simulink model "TEModel_random"  (Simulink 8.3)
settings: Solver=ode1  SolverMode=SingleTasking  StartTime=0.0  StopTime=72  FixedStep=Ts_base  MaxStep=Ts_base  MinStep=1e-6  RelTol=1e-6
PreLoadFcn:
  | initModel
StopFcn:
  | TEplot
undefined symbols (not defined in the file): Ts_base, Ts_save
libraries: VAlib x28, TElib x18
(part 9 of 9)

== system TEModel_random/TE Plant/xmeas atk block/xmeas3 attack controller/Attack Type Controller/interval forward controller ==
  normal : Inport
  faked : Inport  Port=2
  Impuls : VAlib/Impuls  amplitude=1  duration=duration  delay=start
  Switch : Switch  Criteria=u2 > Threshold
  output : Outport
  wires:
  faked/1 -> Switch/1
  normal/1 -> Switch/3
  Impuls/1 -> Switch/2
  Switch/1 -> output/1

== system TEModel_random/TE Plant/xmeas atk block/xmeas3 attack controller/Attack Type Controller/normal forward controller ==
  normal : Inport
  faked : Inport  Port=2
  Terminator : Terminator
  output : Outport
  wires:
  normal/1 -> output/1
  faked/1 -> Terminator/1

== system TEModel_random/TE Plant/xmeas atk block/xmeas3 attack controller/Attack Type Controller/periodical forward controller ==
  normal : Inport
  faked : Inport  Port=2
  Pulse Generator : DiscretePulseGenerator  PulseType=Time based  Period=duration + start  PulseWidth=100*duration/(duration + start)  PhaseDelay=start
  Switch : Switch  Criteria=u2 > Threshold
  output : Outport
  wires:
  faked/1 -> Switch/1
  normal/1 -> Switch/3
  Pulse Generator/1 -> Switch/2
  Switch/1 -> output/1

== system TEModel_random/TE Plant/xmeas atk block/xmeas3 attack controller/Attack Type Controller/step forward controller ==
  normal : Inport
  faked : Inport  Port=2
  Step : Step  Time=start  SampleTime=0
  Switch : Switch  Criteria=u2 > Threshold
  output : Outport
  wires:
  faked/1 -> Switch/1
  normal/1 -> Switch/3
  Step/1 -> Switch/2
  Switch/1 -> output/1

== system TEModel_random/TE Plant/xmeas atk block/xmeas31 attack controller/Attack Type Controller/interval forward controller ==
  normal : Inport
  faked : Inport  Port=2
  Impuls : VAlib/Impuls  amplitude=1  duration=duration  delay=start
  Switch : Switch  Criteria=u2 > Threshold
  output : Outport
  wires:
  faked/1 -> Switch/1
  normal/1 -> Switch/3
  Impuls/1 -> Switch/2
  Switch/1 -> output/1

== system TEModel_random/TE Plant/xmeas atk block/xmeas31 attack controller/Attack Type Controller/normal forward controller ==
  normal : Inport
  faked : Inport  Port=2
  Terminator : Terminator
  output : Outport
  wires:
  normal/1 -> output/1
  faked/1 -> Terminator/1

== system TEModel_random/TE Plant/xmeas atk block/xmeas31 attack controller/Attack Type Controller/periodical forward controller ==
  normal : Inport
  faked : Inport  Port=2
  Pulse Generator : DiscretePulseGenerator  PulseType=Time based  Period=duration + start  PulseWidth=100*duration/(duration + start)  PhaseDelay=start
  Switch : Switch  Criteria=u2 > Threshold
  output : Outport
  wires:
  faked/1 -> Switch/1
  normal/1 -> Switch/3
  Pulse Generator/1 -> Switch/2
  Switch/1 -> output/1

== system TEModel_random/TE Plant/xmeas atk block/xmeas31 attack controller/Attack Type Controller/step forward controller ==
  normal : Inport
  faked : Inport  Port=2
  Step : Step  Time=start  SampleTime=0
  Switch : Switch  Criteria=u2 > Threshold
  output : Outport
  wires:
  faked/1 -> Switch/1
  normal/1 -> Switch/3
  Step/1 -> Switch/2
  Switch/1 -> output/1

== system TEModel_random/TE Plant/xmeas atk block/xmeas4 attack controller/Attack Type Controller/interval forward controller ==
  normal : Inport
  faked : Inport  Port=2
  Impuls : VAlib/Impuls  amplitude=1  duration=duration  delay=start
  Switch : Switch  Criteria=u2 > Threshold
  output : Outport
  wires:
  faked/1 -> Switch/1
  normal/1 -> Switch/3
  Impuls/1 -> Switch/2
  Switch/1 -> output/1

== system TEModel_random/TE Plant/xmeas atk block/xmeas4 attack controller/Attack Type Controller/normal forward controller ==
  normal : Inport
  faked : Inport  Port=2
  Terminator : Terminator
  output : Outport
  wires:
  normal/1 -> output/1
  faked/1 -> Terminator/1

== system TEModel_random/TE Plant/xmeas atk block/xmeas4 attack controller/Attack Type Controller/periodical forward controller ==
  normal : Inport
  faked : Inport  Port=2
  Pulse Generator : DiscretePulseGenerator  PulseType=Time based  Period=duration + start  PulseWidth=100*duration/(duration + start)  PhaseDelay=start
  Switch : Switch  Criteria=u2 > Threshold
  output : Outport
  wires:
  faked/1 -> Switch/1
  normal/1 -> Switch/3
  Pulse Generator/1 -> Switch/2
  Switch/1 -> output/1

== system TEModel_random/TE Plant/xmeas atk block/xmeas4 attack controller/Attack Type Controller/step forward controller ==
  normal : Inport
  faked : Inport  Port=2
  Step : Step  Time=start  SampleTime=0
  Switch : Switch  Criteria=u2 > Threshold
  output : Outport
  wires:
  faked/1 -> Switch/1
  normal/1 -> Switch/3
  Step/1 -> Switch/2
  Switch/1 -> output/1

== system TEModel_random/TE Plant/xmeas atk block/xmeas40 attack controller/Attack Type Controller/interval forward controller ==
  normal : Inport
  faked : Inport  Port=2
  Impuls : VAlib/Impuls  amplitude=1  duration=duration  delay=start
  Switch : Switch  Criteria=u2 > Threshold
  output : Outport
  wires:
  faked/1 -> Switch/1
  normal/1 -> Switch/3
  Impuls/1 -> Switch/2
  Switch/1 -> output/1

== system TEModel_random/TE Plant/xmeas atk block/xmeas40 attack controller/Attack Type Controller/normal forward controller ==
  normal : Inport
  faked : Inport  Port=2
  Terminator : Terminator
  output : Outport
  wires:
  normal/1 -> output/1
  faked/1 -> Terminator/1

== system TEModel_random/TE Plant/xmeas atk block/xmeas40 attack controller/Attack Type Controller/periodical forward controller ==
  normal : Inport
  faked : Inport  Port=2
  Pulse Generator : DiscretePulseGenerator  PulseType=Time based  Period=duration + start  PulseWidth=100*duration/(duration + start)  PhaseDelay=start
  Switch : Switch  Criteria=u2 > Threshold
  output : Outport
  wires:
  faked/1 -> Switch/1
  normal/1 -> Switch/3
  Pulse Generator/1 -> Switch/2
  Switch/1 -> output/1

== system TEModel_random/TE Plant/xmeas atk block/xmeas40 attack controller/Attack Type Controller/step forward controller ==
  normal : Inport
  faked : Inport  Port=2
  Step : Step  Time=start  SampleTime=0
  Switch : Switch  Criteria=u2 > Threshold
  output : Outport
  wires:
  faked/1 -> Switch/1
  normal/1 -> Switch/3
  Step/1 -> Switch/2
  Switch/1 -> output/1

== system TEModel_random/TE Plant/xmeas atk block/xmeas5 attack controller/Attack Type Controller/interval forward controller ==
  normal : Inport
  faked : Inport  Port=2
  Impuls : VAlib/Impuls  amplitude=1  duration=duration  delay=start
  Switch : Switch  Criteria=u2 > Threshold
  output : Outport
  wires:
  faked/1 -> Switch/1
  normal/1 -> Switch/3
  Impuls/1 -> Switch/2
  Switch/1 -> output/1

== system TEModel_random/TE Plant/xmeas atk block/xmeas5 attack controller/Attack Type Controller/normal forward controller ==
  normal : Inport
  faked : Inport  Port=2
  Terminator : Terminator
  output : Outport
  wires:
  normal/1 -> output/1
  faked/1 -> Terminator/1

== system TEModel_random/TE Plant/xmeas atk block/xmeas5 attack controller/Attack Type Controller/periodical forward controller ==
  normal : Inport
  faked : Inport  Port=2
  Pulse Generator : DiscretePulseGenerator  PulseType=Time based  Period=duration + start  PulseWidth=100*duration/(duration + start)  PhaseDelay=start
  Switch : Switch  Criteria=u2 > Threshold
  output : Outport
  wires:
  faked/1 -> Switch/1
  normal/1 -> Switch/3
  Pulse Generator/1 -> Switch/2
  Switch/1 -> output/1

== system TEModel_random/TE Plant/xmeas atk block/xmeas5 attack controller/Attack Type Controller/step forward controller ==
  normal : Inport
  faked : Inport  Port=2
  Step : Step  Time=start  SampleTime=0
  Switch : Switch  Criteria=u2 > Threshold
  output : Outport
  wires:
  faked/1 -> Switch/1
  normal/1 -> Switch/3
  Step/1 -> Switch/2
  Switch/1 -> output/1

== system TEModel_random/TE Plant/xmeas atk block/xmeas7 attack controller/Attack Type Controller/interval forward controller ==
  normal : Inport
  faked : Inport  Port=2
  Impuls : VAlib/Impuls  amplitude=1  duration=duration  delay=start
  Switch : Switch  Criteria=u2 > Threshold
  output : Outport
  wires:
  faked/1 -> Switch/1
  normal/1 -> Switch/3
  Impuls/1 -> Switch/2
  Switch/1 -> output/1

== system TEModel_random/TE Plant/xmeas atk block/xmeas7 attack controller/Attack Type Controller/normal forward controller ==
  normal : Inport
  faked : Inport  Port=2
  Terminator : Terminator
  output : Outport
  wires:
  normal/1 -> output/1
  faked/1 -> Terminator/1

== system TEModel_random/TE Plant/xmeas atk block/xmeas7 attack controller/Attack Type Controller/periodical forward controller ==
  normal : Inport
  faked : Inport  Port=2
  Pulse Generator : DiscretePulseGenerator  PulseType=Time based  Period=duration + start  PulseWidth=100*duration/(duration + start)  PhaseDelay=start
  Switch : Switch  Criteria=u2 > Threshold
  output : Outport
  wires:
  faked/1 -> Switch/1
  normal/1 -> Switch/3
  Pulse Generator/1 -> Switch/2
  Switch/1 -> output/1

== system TEModel_random/TE Plant/xmeas atk block/xmeas7 attack controller/Attack Type Controller/step forward controller ==
  normal : Inport
  faked : Inport  Port=2
  Step : Step  Time=start  SampleTime=0
  Switch : Switch  Criteria=u2 > Threshold
  output : Outport
  wires:
  faked/1 -> Switch/1
  normal/1 -> Switch/3
  Step/1 -> Switch/2
  Switch/1 -> output/1

== system TEModel_random/TE Plant/xmeas atk block/xmeas8 attack controller/Attack Type Controller/interval forward controller ==
  normal : Inport
  faked : Inport  Port=2
  Impuls : VAlib/Impuls  amplitude=1  duration=duration  delay=start
  Switch : Switch  Criteria=u2 > Threshold
  output : Outport
  wires:
  faked/1 -> Switch/1
  normal/1 -> Switch/3
  Impuls/1 -> Switch/2
  Switch/1 -> output/1

== system TEModel_random/TE Plant/xmeas atk block/xmeas8 attack controller/Attack Type Controller/normal forward controller ==
  normal : Inport
  faked : Inport  Port=2
  Terminator : Terminator
  output : Outport
  wires:
  normal/1 -> output/1
  faked/1 -> Terminator/1

== system TEModel_random/TE Plant/xmeas atk block/xmeas8 attack controller/Attack Type Controller/periodical forward controller ==
  normal : Inport
  faked : Inport  Port=2
  Pulse Generator : DiscretePulseGenerator  PulseType=Time based  Period=duration + start  PulseWidth=100*duration/(duration + start)  PhaseDelay=start
  Switch : Switch  Criteria=u2 > Threshold
  output : Outport
  wires:
  faked/1 -> Switch/1
  normal/1 -> Switch/3
  Pulse Generator/1 -> Switch/2
  Switch/1 -> output/1

== system TEModel_random/TE Plant/xmeas atk block/xmeas8 attack controller/Attack Type Controller/step forward controller ==
  normal : Inport
  faked : Inport  Port=2
  Step : Step  Time=start  SampleTime=0
  Switch : Switch  Criteria=u2 > Threshold
  output : Outport
  wires:
  faked/1 -> Switch/1
  normal/1 -> Switch/3
  Step/1 -> Switch/2
  Switch/1 -> output/1

== system TEModel_random/TE Plant/xmeas atk block/xmeas9 attack controller/Attack Type Controller/interval forward controller ==
  normal : Inport
  faked : Inport  Port=2
  Impuls : VAlib/Impuls  amplitude=1  duration=duration  delay=start
  Switch : Switch  Criteria=u2 > Threshold
  output : Outport
  wires:
  faked/1 -> Switch/1
  normal/1 -> Switch/3
  Impuls/1 -> Switch/2
  Switch/1 -> output/1

== system TEModel_random/TE Plant/xmeas atk block/xmeas9 attack controller/Attack Type Controller/normal forward controller ==
  normal : Inport
  faked : Inport  Port=2
  Terminator : Terminator
  output : Outport
  wires:
  normal/1 -> output/1
  faked/1 -> Terminator/1

== system TEModel_random/TE Plant/xmeas atk block/xmeas9 attack controller/Attack Type Controller/periodical forward controller ==
  normal : Inport
  faked : Inport  Port=2
  Pulse Generator : DiscretePulseGenerator  PulseType=Time based  Period=duration + start  PulseWidth=100*duration/(duration + start)  PhaseDelay=start
  Switch : Switch  Criteria=u2 > Threshold
  output : Outport
  wires:
  faked/1 -> Switch/1
  normal/1 -> Switch/3
  Pulse Generator/1 -> Switch/2
  Switch/1 -> output/1

== system TEModel_random/TE Plant/xmeas atk block/xmeas9 attack controller/Attack Type Controller/step forward controller ==
  normal : Inport
  faked : Inport  Port=2
  Step : Step  Time=start  SampleTime=0
  Switch : Switch  Criteria=u2 > Threshold
  output : Outport
  wires:
  faked/1 -> Switch/1
  normal/1 -> Switch/3
  Step/1 -> Switch/2
  Switch/1 -> output/1

== system TEModel_random/TE Plant/xmv atk block/xmv1 attack controller/Attack Type Controller/interval forward controller ==
  normal : Inport
  faked : Inport  Port=2
  Impuls : VAlib/Impuls  amplitude=1  duration=duration  delay=start
  Switch : Switch  Criteria=u2 > Threshold
  output : Outport
  wires:
  faked/1 -> Switch/1
  normal/1 -> Switch/3
  Impuls/1 -> Switch/2
  Switch/1 -> output/1

== system TEModel_random/TE Plant/xmv atk block/xmv1 attack controller/Attack Type Controller/normal forward controller ==
  normal : Inport
  faked : Inport  Port=2
  Terminator : Terminator
  output : Outport
  wires:
  normal/1 -> output/1
  faked/1 -> Terminator/1

== system TEModel_random/TE Plant/xmv atk block/xmv1 attack controller/Attack Type Controller/periodical forward controller ==
  normal : Inport
  faked : Inport  Port=2
  Pulse Generator : DiscretePulseGenerator  PulseType=Time based  Period=duration + start  PulseWidth=100*duration/(duration + start)  PhaseDelay=start
  Switch : Switch  Criteria=u2 > Threshold
  output : Outport
  wires:
  faked/1 -> Switch/1
  normal/1 -> Switch/3
  Pulse Generator/1 -> Switch/2
  Switch/1 -> output/1

== system TEModel_random/TE Plant/xmv atk block/xmv1 attack controller/Attack Type Controller/step forward controller ==
  normal : Inport
  faked : Inport  Port=2
  Step : Step  Time=start  SampleTime=0
  Switch : Switch  Criteria=u2 > Threshold
  output : Outport
  wires:
  faked/1 -> Switch/1
  normal/1 -> Switch/3
  Step/1 -> Switch/2
  Switch/1 -> output/1

== system TEModel_random/TE Plant/xmv atk block/xmv10 attack controller/Attack Type Controller/interval forward controller ==
  normal : Inport
  faked : Inport  Port=2
  Impuls : VAlib/Impuls  amplitude=1  duration=duration  delay=start
  Switch : Switch  Criteria=u2 > Threshold
  output : Outport
  wires:
  faked/1 -> Switch/1
  normal/1 -> Switch/3
  Impuls/1 -> Switch/2
  Switch/1 -> output/1

== system TEModel_random/TE Plant/xmv atk block/xmv10 attack controller/Attack Type Controller/normal forward controller ==
  normal : Inport
  faked : Inport  Port=2
  Terminator : Terminator
  output : Outport
  wires:
  normal/1 -> output/1
  faked/1 -> Terminator/1

== system TEModel_random/TE Plant/xmv atk block/xmv10 attack controller/Attack Type Controller/periodical forward controller ==
  normal : Inport
  faked : Inport  Port=2
  Pulse Generator : DiscretePulseGenerator  PulseType=Time based  Period=duration + start  PulseWidth=100*duration/(duration + start)  PhaseDelay=start
  Switch : Switch  Criteria=u2 > Threshold
  output : Outport
  wires:
  faked/1 -> Switch/1
  normal/1 -> Switch/3
  Pulse Generator/1 -> Switch/2
  Switch/1 -> output/1

== system TEModel_random/TE Plant/xmv atk block/xmv10 attack controller/Attack Type Controller/step forward controller ==
  normal : Inport
  faked : Inport  Port=2
  Step : Step  Time=start  SampleTime=0
  Switch : Switch  Criteria=u2 > Threshold
  output : Outport
  wires:
  faked/1 -> Switch/1
  normal/1 -> Switch/3
  Step/1 -> Switch/2
  Switch/1 -> output/1

== system TEModel_random/TE Plant/xmv atk block/xmv11 attack controller/Attack Type Controller/interval forward controller ==
  normal : Inport
  faked : Inport  Port=2
  Impuls : VAlib/Impuls  amplitude=1  duration=duration  delay=start
  Switch : Switch  Criteria=u2 > Threshold
  output : Outport
  wires:
  faked/1 -> Switch/1
  normal/1 -> Switch/3
  Impuls/1 -> Switch/2
  Switch/1 -> output/1

== system TEModel_random/TE Plant/xmv atk block/xmv11 attack controller/Attack Type Controller/normal forward controller ==
  normal : Inport
  faked : Inport  Port=2
  Terminator : Terminator
  output : Outport
  wires:
  normal/1 -> output/1
  faked/1 -> Terminator/1

== system TEModel_random/TE Plant/xmv atk block/xmv11 attack controller/Attack Type Controller/periodical forward controller ==
  normal : Inport
  faked : Inport  Port=2
  Pulse Generator : DiscretePulseGenerator  PulseType=Time based  Period=duration + start  PulseWidth=100*duration/(duration + start)  PhaseDelay=start
  Switch : Switch  Criteria=u2 > Threshold
  output : Outport
  wires:
  faked/1 -> Switch/1
  normal/1 -> Switch/3
  Pulse Generator/1 -> Switch/2
  Switch/1 -> output/1

== system TEModel_random/TE Plant/xmv atk block/xmv11 attack controller/Attack Type Controller/step forward controller ==
  normal : Inport
  faked : Inport  Port=2
  Step : Step  Time=start  SampleTime=0
  Switch : Switch  Criteria=u2 > Threshold
  output : Outport
  wires:
  faked/1 -> Switch/1
  normal/1 -> Switch/3
  Step/1 -> Switch/2
  Switch/1 -> output/1

== system TEModel_random/TE Plant/xmv atk block/xmv12 attack controller/Attack Type Controller/interval forward controller ==
  normal : Inport
  faked : Inport  Port=2
  Impuls : VAlib/Impuls  amplitude=1  duration=duration  delay=start
  Switch : Switch  Criteria=u2 > Threshold
  output : Outport
  wires:
  faked/1 -> Switch/1
  normal/1 -> Switch/3
  Impuls/1 -> Switch/2
  Switch/1 -> output/1

== system TEModel_random/TE Plant/xmv atk block/xmv12 attack controller/Attack Type Controller/normal forward controller ==
  normal : Inport
  faked : Inport  Port=2
  Terminator : Terminator
  output : Outport
  wires:
  normal/1 -> output/1
  faked/1 -> Terminator/1

== system TEModel_random/TE Plant/xmv atk block/xmv12 attack controller/Attack Type Controller/periodical forward controller ==
  normal : Inport
  faked : Inport  Port=2
  Pulse Generator : DiscretePulseGenerator  PulseType=Time based  Period=duration + start  PulseWidth=100*duration/(duration + start)  PhaseDelay=start
  Switch : Switch  Criteria=u2 > Threshold
  output : Outport
  wires:
  faked/1 -> Switch/1
  normal/1 -> Switch/3
  Pulse Generator/1 -> Switch/2
  Switch/1 -> output/1

== system TEModel_random/TE Plant/xmv atk block/xmv12 attack controller/Attack Type Controller/step forward controller ==
  normal : Inport
  faked : Inport  Port=2
  Step : Step  Time=start  SampleTime=0
  Switch : Switch  Criteria=u2 > Threshold
  output : Outport
  wires:
  faked/1 -> Switch/1
  normal/1 -> Switch/3
  Step/1 -> Switch/2
  Switch/1 -> output/1

== system TEModel_random/TE Plant/xmv atk block/xmv2 attack controller/Attack Type Controller/interval forward controller ==
  normal : Inport
  faked : Inport  Port=2
  Impuls : VAlib/Impuls  amplitude=1  duration=duration  delay=start
  Switch : Switch  Criteria=u2 > Threshold
  output : Outport
  wires:
  faked/1 -> Switch/1
  normal/1 -> Switch/3
  Impuls/1 -> Switch/2
  Switch/1 -> output/1

== system TEModel_random/TE Plant/xmv atk block/xmv2 attack controller/Attack Type Controller/normal forward controller ==
  normal : Inport
  faked : Inport  Port=2
  Terminator : Terminator
  output : Outport
  wires:
  normal/1 -> output/1
  faked/1 -> Terminator/1

== system TEModel_random/TE Plant/xmv atk block/xmv2 attack controller/Attack Type Controller/periodical forward controller ==
  normal : Inport
  faked : Inport  Port=2
  Pulse Generator : DiscretePulseGenerator  PulseType=Time based  Period=duration + start  PulseWidth=100*duration/(duration + start)  PhaseDelay=start
  Switch : Switch  Criteria=u2 > Threshold
  output : Outport
  wires:
  faked/1 -> Switch/1
  normal/1 -> Switch/3
  Pulse Generator/1 -> Switch/2
  Switch/1 -> output/1

== system TEModel_random/TE Plant/xmv atk block/xmv2 attack controller/Attack Type Controller/step forward controller ==
  normal : Inport
  faked : Inport  Port=2
  Step : Step  Time=start  SampleTime=0
  Switch : Switch  Criteria=u2 > Threshold
  output : Outport
  wires:
  faked/1 -> Switch/1
  normal/1 -> Switch/3
  Step/1 -> Switch/2
  Switch/1 -> output/1

== system TEModel_random/TE Plant/xmv atk block/xmv3 attack controller/Attack Type Controller/interval forward controller ==
  normal : Inport
  faked : Inport  Port=2
  Impuls : VAlib/Impuls  amplitude=1  duration=duration  delay=start
  Switch : Switch  Criteria=u2 > Threshold
  output : Outport
  wires:
  faked/1 -> Switch/1
  normal/1 -> Switch/3
  Impuls/1 -> Switch/2
  Switch/1 -> output/1

== system TEModel_random/TE Plant/xmv atk block/xmv3 attack controller/Attack Type Controller/normal forward controller ==
  normal : Inport
  faked : Inport  Port=2
  Terminator : Terminator
  output : Outport
  wires:
  normal/1 -> output/1
  faked/1 -> Terminator/1

== system TEModel_random/TE Plant/xmv atk block/xmv3 attack controller/Attack Type Controller/periodical forward controller ==
  normal : Inport
  faked : Inport  Port=2
  Pulse Generator : DiscretePulseGenerator  PulseType=Time based  Period=duration + start  PulseWidth=100*duration/(duration + start)  PhaseDelay=start
  Switch : Switch  Criteria=u2 > Threshold
  output : Outport
  wires:
  faked/1 -> Switch/1
  normal/1 -> Switch/3
  Pulse Generator/1 -> Switch/2
  Switch/1 -> output/1

== system TEModel_random/TE Plant/xmv atk block/xmv3 attack controller/Attack Type Controller/step forward controller ==
  normal : Inport
  faked : Inport  Port=2
  Step : Step  Time=start  SampleTime=0
  Switch : Switch  Criteria=u2 > Threshold
  output : Outport
  wires:
  faked/1 -> Switch/1
  normal/1 -> Switch/3
  Step/1 -> Switch/2
  Switch/1 -> output/1

== system TEModel_random/TE Plant/xmv atk block/xmv4 attack controller/Attack Type Controller/interval forward controller ==
  normal : Inport
  faked : Inport  Port=2
  Impuls : VAlib/Impuls  amplitude=1  duration=duration  delay=start
  Switch : Switch  Criteria=u2 > Threshold
  output : Outport
  wires:
  faked/1 -> Switch/1
  normal/1 -> Switch/3
  Impuls/1 -> Switch/2
  Switch/1 -> output/1

== system TEModel_random/TE Plant/xmv atk block/xmv4 attack controller/Attack Type Controller/normal forward controller ==
  normal : Inport
  faked : Inport  Port=2
  Terminator : Terminator
  output : Outport
  wires:
  normal/1 -> output/1
  faked/1 -> Terminator/1

== system TEModel_random/TE Plant/xmv atk block/xmv4 attack controller/Attack Type Controller/periodical forward controller ==
  normal : Inport
  faked : Inport  Port=2
  Pulse Generator : DiscretePulseGenerator  PulseType=Time based  Period=duration + start  PulseWidth=100*duration/(duration + start)  PhaseDelay=start
  Switch : Switch  Criteria=u2 > Threshold
  output : Outport
  wires:
  faked/1 -> Switch/1
  normal/1 -> Switch/3
  Pulse Generator/1 -> Switch/2
  Switch/1 -> output/1

== system TEModel_random/TE Plant/xmv atk block/xmv4 attack controller/Attack Type Controller/step forward controller ==
  normal : Inport
  faked : Inport  Port=2
  Step : Step  Time=start  SampleTime=0
  Switch : Switch  Criteria=u2 > Threshold
  output : Outport
  wires:
  faked/1 -> Switch/1
  normal/1 -> Switch/3
  Step/1 -> Switch/2
  Switch/1 -> output/1

== system TEModel_random/TE Plant/xmv atk block/xmv5 attack controller/Attack Type Controller/interval forward controller ==
  normal : Inport
  faked : Inport  Port=2
  Impuls : VAlib/Impuls  amplitude=1  duration=duration  delay=start
  Switch : Switch  Criteria=u2 > Threshold
  output : Outport
  wires:
  faked/1 -> Switch/1
  normal/1 -> Switch/3
  Impuls/1 -> Switch/2
  Switch/1 -> output/1

== system TEModel_random/TE Plant/xmv atk block/xmv5 attack controller/Attack Type Controller/normal forward controller ==
  normal : Inport
  faked : Inport  Port=2
  Terminator : Terminator
  output : Outport
  wires:
  normal/1 -> output/1
  faked/1 -> Terminator/1

== system TEModel_random/TE Plant/xmv atk block/xmv5 attack controller/Attack Type Controller/periodical forward controller ==
  normal : Inport
  faked : Inport  Port=2
  Pulse Generator : DiscretePulseGenerator  PulseType=Time based  Period=duration + start  PulseWidth=100*duration/(duration + start)  PhaseDelay=start
  Switch : Switch  Criteria=u2 > Threshold
  output : Outport
  wires:
  faked/1 -> Switch/1
  normal/1 -> Switch/3
  Pulse Generator/1 -> Switch/2
  Switch/1 -> output/1

== system TEModel_random/TE Plant/xmv atk block/xmv5 attack controller/Attack Type Controller/step forward controller ==
  normal : Inport
  faked : Inport  Port=2
  Step : Step  Time=start  SampleTime=0
  Switch : Switch  Criteria=u2 > Threshold
  output : Outport
  wires:
  faked/1 -> Switch/1
  normal/1 -> Switch/3
  Step/1 -> Switch/2
  Switch/1 -> output/1

== system TEModel_random/TE Plant/xmv atk block/xmv6 attack controller/Attack Type Controller/interval forward controller ==
  normal : Inport
  faked : Inport  Port=2
  Impuls : VAlib/Impuls  amplitude=1  duration=duration  delay=start
  Switch : Switch  Criteria=u2 > Threshold
  output : Outport
  wires:
  faked/1 -> Switch/1
  normal/1 -> Switch/3
  Impuls/1 -> Switch/2
  Switch/1 -> output/1

== system TEModel_random/TE Plant/xmv atk block/xmv6 attack controller/Attack Type Controller/normal forward controller ==
  normal : Inport
  faked : Inport  Port=2
  Terminator : Terminator
  output : Outport
  wires:
  normal/1 -> output/1
  faked/1 -> Terminator/1

== system TEModel_random/TE Plant/xmv atk block/xmv6 attack controller/Attack Type Controller/periodical forward controller ==
  normal : Inport
  faked : Inport  Port=2
  Pulse Generator : DiscretePulseGenerator  PulseType=Time based  Period=duration + start  PulseWidth=100*duration/(duration + start)  PhaseDelay=start
  Switch : Switch  Criteria=u2 > Threshold
  output : Outport
  wires:
  faked/1 -> Switch/1
  normal/1 -> Switch/3
  Pulse Generator/1 -> Switch/2
  Switch/1 -> output/1

== system TEModel_random/TE Plant/xmv atk block/xmv6 attack controller/Attack Type Controller/step forward controller ==
  normal : Inport
  faked : Inport  Port=2
  Step : Step  Time=start  SampleTime=0
  Switch : Switch  Criteria=u2 > Threshold
  output : Outport
  wires:
  faked/1 -> Switch/1
  normal/1 -> Switch/3
  Step/1 -> Switch/2
  Switch/1 -> output/1

== system TEModel_random/TE Plant/xmv atk block/xmv7 attack controller/Attack Type Controller/interval forward controller ==
  normal : Inport
  faked : Inport  Port=2
  Impuls : VAlib/Impuls  amplitude=1  duration=duration  delay=start
  Switch : Switch  Criteria=u2 > Threshold
  output : Outport
  wires:
  faked/1 -> Switch/1
  normal/1 -> Switch/3
  Impuls/1 -> Switch/2
  Switch/1 -> output/1

== system TEModel_random/TE Plant/xmv atk block/xmv7 attack controller/Attack Type Controller/normal forward controller ==
  normal : Inport
  faked : Inport  Port=2
  Terminator : Terminator
  output : Outport
  wires:
  normal/1 -> output/1
  faked/1 -> Terminator/1

== system TEModel_random/TE Plant/xmv atk block/xmv7 attack controller/Attack Type Controller/periodical forward controller ==
  normal : Inport
  faked : Inport  Port=2
  Pulse Generator : DiscretePulseGenerator  PulseType=Time based  Period=duration + start  PulseWidth=100*duration/(duration + start)  PhaseDelay=start
  Switch : Switch  Criteria=u2 > Threshold
  output : Outport
  wires:
  faked/1 -> Switch/1
  normal/1 -> Switch/3
  Pulse Generator/1 -> Switch/2
  Switch/1 -> output/1

== system TEModel_random/TE Plant/xmv atk block/xmv7 attack controller/Attack Type Controller/step forward controller ==
  normal : Inport
  faked : Inport  Port=2
  Step : Step  Time=start  SampleTime=0
  Switch : Switch  Criteria=u2 > Threshold
  output : Outport
  wires:
  faked/1 -> Switch/1
  normal/1 -> Switch/3
  Step/1 -> Switch/2
  Switch/1 -> output/1

== system TEModel_random/TE Plant/xmv atk block/xmv8 attack controller/Attack Type Controller/interval forward controller ==
  normal : Inport
  faked : Inport  Port=2
  Impuls : VAlib/Impuls  amplitude=1  duration=duration  delay=start
  Switch : Switch  Criteria=u2 > Threshold
  output : Outport
  wires:
  faked/1 -> Switch/1
  normal/1 -> Switch/3
  Impuls/1 -> Switch/2
  Switch/1 -> output/1

== system TEModel_random/TE Plant/xmv atk block/xmv8 attack controller/Attack Type Controller/normal forward controller ==
  normal : Inport
  faked : Inport  Port=2
  Terminator : Terminator
  output : Outport
  wires:
  normal/1 -> output/1
  faked/1 -> Terminator/1

== system TEModel_random/TE Plant/xmv atk block/xmv8 attack controller/Attack Type Controller/periodical forward controller ==
  normal : Inport
  faked : Inport  Port=2
  Pulse Generator : DiscretePulseGenerator  PulseType=Time based  Period=duration + start  PulseWidth=100*duration/(duration + start)  PhaseDelay=start
  Switch : Switch  Criteria=u2 > Threshold
  output : Outport
  wires:
  faked/1 -> Switch/1
  normal/1 -> Switch/3
  Pulse Generator/1 -> Switch/2
  Switch/1 -> output/1

== system TEModel_random/TE Plant/xmv atk block/xmv8 attack controller/Attack Type Controller/step forward controller ==
  normal : Inport
  faked : Inport  Port=2
  Step : Step  Time=start  SampleTime=0
  Switch : Switch  Criteria=u2 > Threshold
  output : Outport
  wires:
  faked/1 -> Switch/1
  normal/1 -> Switch/3
  Step/1 -> Switch/2
  Switch/1 -> output/1

== system TEModel_random/TE Plant/xmv atk block/xmv9 attack controller/Attack Type Controller/interval forward controller ==
  normal : Inport
  faked : Inport  Port=2
  Impuls : VAlib/Impuls  amplitude=1  duration=duration  delay=start
  Switch : Switch  Criteria=u2 > Threshold
  output : Outport
  wires:
  faked/1 -> Switch/1
  normal/1 -> Switch/3
  Impuls/1 -> Switch/2
  Switch/1 -> output/1

== system TEModel_random/TE Plant/xmv atk block/xmv9 attack controller/Attack Type Controller/normal forward controller ==
  normal : Inport
  faked : Inport  Port=2
  Terminator : Terminator
  output : Outport
  wires:
  normal/1 -> output/1
  faked/1 -> Terminator/1

== system TEModel_random/TE Plant/xmv atk block/xmv9 attack controller/Attack Type Controller/periodical forward controller ==
  normal : Inport
  faked : Inport  Port=2
  Pulse Generator : DiscretePulseGenerator  PulseType=Time based  Period=duration + start  PulseWidth=100*duration/(duration + start)  PhaseDelay=start
  Switch : Switch  Criteria=u2 > Threshold
  output : Outport
  wires:
  faked/1 -> Switch/1
  normal/1 -> Switch/3
  Pulse Generator/1 -> Switch/2
  Switch/1 -> output/1

== system TEModel_random/TE Plant/xmv atk block/xmv9 attack controller/Attack Type Controller/step forward controller ==
  normal : Inport
  faked : Inport  Port=2
  Step : Step  Time=start  SampleTime=0
  Switch : Switch  Criteria=u2 > Threshold
  output : Outport
  wires:
  faked/1 -> Switch/1
  normal/1 -> Switch/3
  Step/1 -> Switch/2
  Switch/1 -> output/1

== matlab function TE Plant/MATLAB Function2 ==
  data: u input double; y output double; z input double
function y  = fcn(u,z)

    y=(z/100)*u;
    %plot(t,y);
end
